simulink model "slexModelingServicesExample_org"  (Simulink 10.0)
settings: Solver=FixedStepAuto  StartTime=0.0  StopTime=10.0  RelTol=1e-3  EnableMultiTasking=on
settings Model: Creator=The MathWorks, Inc.  LastModifiedBy=bhisma
settings SolverCC: PositivePriorityOrder=on
settings DataIOCC: SaveFormat=StructureWithTime  ReturnWorkspaceOutputs=on
settings OptimizationCC: DefaultParameterBehavior=Inlined  PassReuseOutputArgsAs=Individual arguments  LifeSpan=auto  MaxStackSize=64  EfficientTunableParamExpr=on
settings DebuggingCC: UnderspecifiedInitializationDetection=Simplified  MergeDetectMultiDrivingBlocksExec=error  ParameterTunabilityLossMsg=error  SFUnexpectedBacktrackingDiag=error  SFNoUnconditionalDefaultTransitionDiag=error  SFExecutionAtInitializationDiag=warning
settings HardwareCC: ProdLargestAtomicInteger=Long  ProdLargestAtomicFloat=Double  ProdIntDivRoundTo=Zero  ProdEndianess=LittleEndian  ProdHWDeviceType=ARM Compatible->ARM Cortex
settings ModelReferenceCC: PropagateSignalLabelsOutOfModel=on
settings SFSimCC: MATLABDynamicMemAlloc=off
settings RTWCC: Description=Embedded Coder  SystemTargetFile=ert.tlc  TemplateMakefile=ert_default_tmf  GenerateReport=on  IncludeHyperlinkInReport=on  LaunchReport=on  GenerateTraceInfo=on  GenerateTraceReport=on  GenerateTraceReportSl=on  GenerateTraceReportSf=on  GenerateTraceReportEml=on
settings CodeAppCC: ForceParamTrailComments=on  IgnoreCustomStorageClasses=off  MaxIdLength=63  OperatorAnnotations=on  SimulinkDataObjDesc=on  SFDataObjDesc=on  InsertBlockDesc=on  StateflowObjectComments=off
settings ERTTargetCC: SupportVariableSizeSignals=on  ERTCustomFileTemplate=example_file_process.tlc
settings ConfigComp: CovMetricSettings=dwe  CovHtmlReporting=off  CovSaveCumulativeToWorkspaceVar=off  CovSaveSingleToWorkspaceVar=off

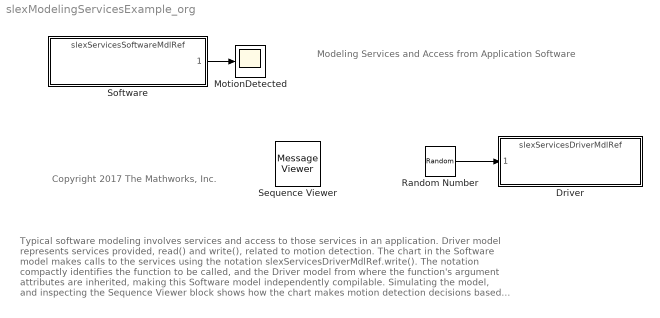
== system slexModelingServicesExample_org ==
  note: Modeling Services and Access from Application Software
  note: Copyright 2017 The Mathworks, Inc.
  note: Typical software modeling involves services and access to those services in an application. Driver model represents services provided, read() and write(), related to motion detection.
      |
      | The chart in the Software model makes calls to the services using the notation slexServicesDriverMdlRef.write(). The notation compactly identifies the function to be called, and the Driver model from where the function's argument attributes are inherited, making this Software model independently compilable.
      |
      | Simulating the model, and inspecting the Sequence Viewer block shows how the chart makes motion detection decisions based on the services.
  Driver : ModelReference  ModelNameDialog=slexServicesDriverMdlRef.slx  SimulationMode=Normal  ScheduleRates=on  ModelReferenceVersion=1.42
  MotionDetected : Scope
  Random Number : RandomNumber  SampleTime=0.1
  Sequence Viewer : MessageViewer  WindowSettings=DataTag0
  Software : ModelReference  ModelNameDialog=slexServicesSoftwareMdlRef.slx  SimulationMode=Normal  ModelReferenceVersion=1.35
  wires:
  Random Number/1 -> Driver/1
  Software/1 -> MotionDetected/1
